simulink model "FiltroPrimerOrdenRealimentado"  (R2017b)
settings: Solver=VariableStepAuto  StartTime=0.0  StopTime=5e-3  RelTol=1e-3
settings Model: Creator=Nicolas Zamora  LastModifiedBy=David
settings CodeAppCC: StateflowObjectComments=on

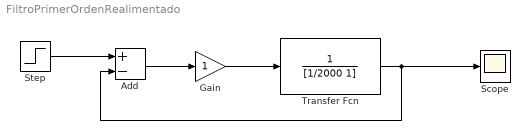
== system FiltroPrimerOrdenRealimentado ==
  Add : Sum  Inputs=+-
  Gain : Gain
  Scope : Scope
  Step : Step  Time=0  After=2  SampleTime=0
  Transfer Fcn : TransferFcn  Denominator=[1/2000 1]
  wires:
  Add/1 -> Gain/1
  Step/1 -> Add/1
  Transfer Fcn/1 -> Scope/1, Add/2
  Gain/1 -> Transfer Fcn/1
